simulink model "model_2_with_mpc"  (R2024a)
settings: Solver=VariableStepAuto  StartTime=0.0  StopTime=5  RelTol=1e-3
values from neighbouring files (symbols this model uses):
  d = 16.5e-2    (= 0.165)    [optParameters.m]
  fM = 8.108e-06    [optParameters.m]
  fw = 0.0047871    [optParameters.m]
  g = 9.8    [optParameters.m]
  JA = 0.00010012    [optParameters.m]
  JB = 0.01862    [optParameters.m]
  JM = 1.1538e-05    [optParameters.m]
  k = 43.8    [optParameters.m]
  kM = 0.0382    [optParameters.m]
  l = -0.02073    [optParameters.m]
  mb = 0.66855    [optParameters.m]
  mw = 53e-3    (= 0.053)    [optParameters.m]
  r = 3.25e-2    (= 0.0325)    [optParameters.m]
  R = 0.2    [load_example_QProblem.m]    (also in lqrandmpc.m = 0.1; optParameters.m = 16.696)
libraries: mpclib x1, aerolibutil x1, sharedutil x1, simulink_extras x1
settings Model: Creator=muham  LastModifiedBy=muham
settings RTWCC: GPUComputeCapability=3.5

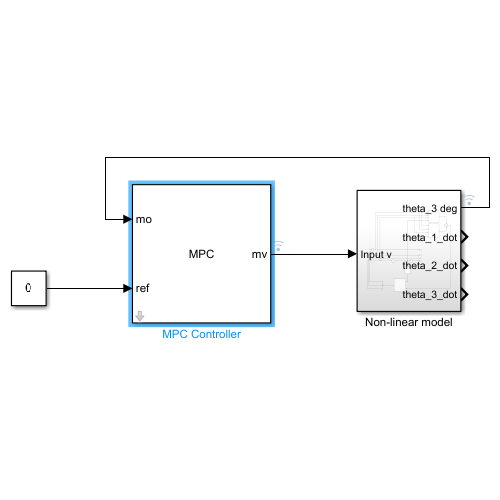
[thumbnail: Simulink's stored preview of the top-level diagram]
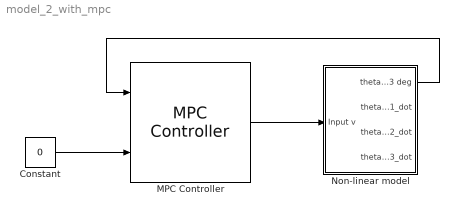
== system model_2_with_mpc ==
  Constant : Constant  Value=0
  MPC Controller : mpclib/MPC Controller  SCDEnableBlockLinearizationSpecification=on  mpcobj=mpc1  is_multiple=0  enable_value=0  return_u0=off  updateMPCinCallerWorkspace=on  md_inport=off  mv_inport=off  uref_inport=off  return_cost=off  return_mvseq=off  return_qpstatus=off  return_xseq=off  return_state=off  return_ovseq=off  state_inport=off  umin_inport=off  umax_inport=off  ymin_inport=off  ymax_inport=off  cc_inport=off  ywt_inport=off  uwt_inport=off  duwt_inport=off  rhoeps_inport=off  pm_inport=off  MaximumP=10  HorizonChoice=FixedHorizon  n_ts=0.01  n_p=40  n_mv=1  n_md=0  n_ud=0  n_mo=1  n_uo=0  BlockDataType=double  SampleTimeInherited=off  switch_inport=off
  Non-linear model : Subsystem
  wires:
  MPC Controller/1 -> Non-linear model/1(Input v)
  Constant/1 -> MPC Controller/2
  Non-linear model/1(theta_3 deg) -> MPC Controller/1

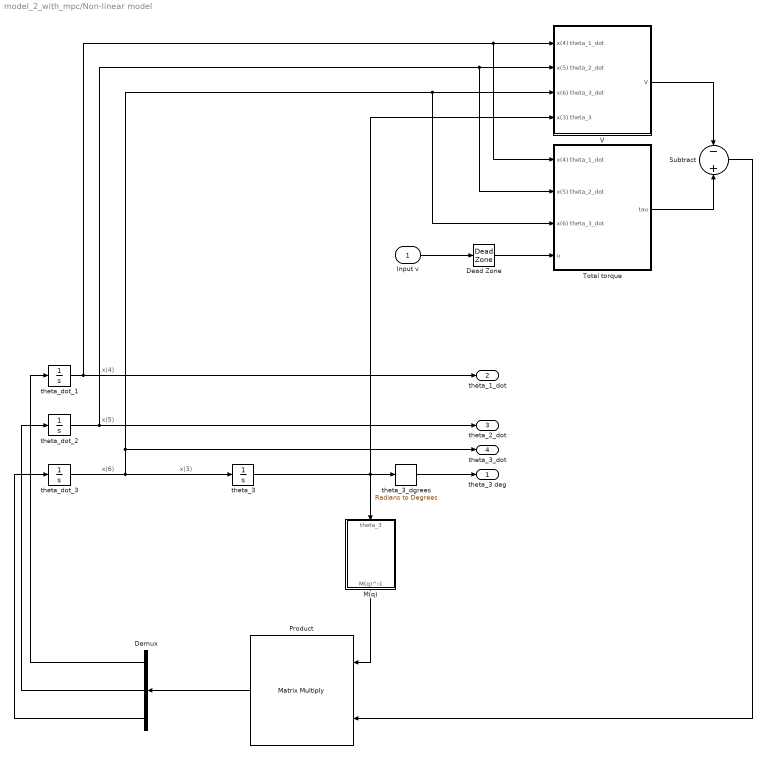
== system model_2_with_mpc/Non-linear model ==
  note: x(3)
  note: x(5)
  note: x(6)
  note: x(4)
  Input v : Inport
  Dead Zone : DeadZone  LowerValue=-1.5  UpperValue=1.5
  Demux : Demux  Outputs=3
  M(q) : Subsystem
  Product : Product  Multiplication=Matrix(*)
  Subtract : Sum  Inputs=-+
  Total torque : Subsystem
  V : Subsystem
  theta_3 : Integrator  WrappedStateUpperValue=pi/2  WrappedStateLowerValue=-pi/2
  theta_3_dgrees : simulink_extras/Transformations/Radians to Degrees
  theta_dot_1 : Integrator
  theta_dot_2 : Integrator
  theta_dot_3 : Integrator
  theta_3 deg : Outport
  theta_1_dot : Outport  Port=2
  theta_2_dot : Outport  Port=3
  theta_3_dot : Outport  Port=4
  wires:
  theta_dot_1/1 -> theta_1_dot/1, V/1(x(4) theta_1_dot), Total torque/1(x(4) theta_1_dot)
  theta_3/1 -> V/4(x(3) theta_3), theta_3_dgrees/1, M(q)/1(theta_3)
  Demux/3 -> theta_dot_3/1
  Demux/1 -> theta_dot_1/1
  Dead Zone/1 -> Total torque/4(u)
  theta_dot_3/1 -> Total torque/3(x(6) theta_3_dot), V/3(x(6) theta_3_dot), theta_3_dot/1, theta_3/1
  theta_3_dgrees/1 -> theta_3 deg/1
  M(q)/1(M(q)^-1) -> Product/1
  Product/1 -> Demux/1
  Subtract/1 -> Product/2
  theta_dot_2/1 -> theta_2_dot/1, V/2(x(5) theta_2_dot), Total torque/2(x(5) theta_2_dot)
  Total torque/1(tau) -> Subtract/2
  Input v/1 -> Dead Zone/1
  Demux/2 -> theta_dot_2/1
  V/1(V) -> Subtract/1

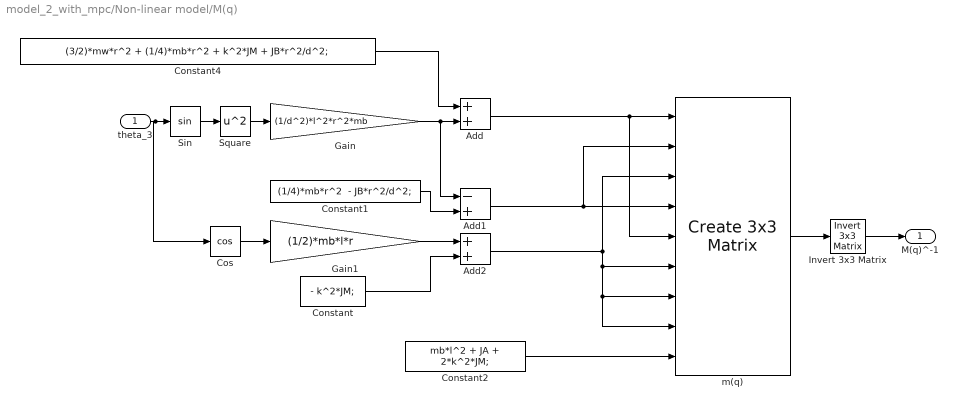
== system model_2_with_mpc/Non-linear model/M(q) ==
  theta_3 : Inport
  Add : Sum
  Add1 : Sum  Inputs=-+
  Add2 : Sum
  Constant : Constant  Value=- k^2*JM;
  Constant1 : Constant  Value="(1/4)*mb*r^2  - JB*r^2/d^2;"
  Constant2 : Constant  Value=mb*l^2 + JA + 2*k^2*JM;
  Constant4 : Constant  Value=(3/2)*mw*r^2 + (1/4)*mb*r^2 + k^2*JM + JB*r^2/d^2;
  Cos : Trigonometry  Operator=cos
  Gain : Gain  Gain=(1/d^2)*l^2*r^2*mb
  Gain1 : Gain  Gain=(1/2)*mb*l*r
  Invert 3x3 Matrix : aerolibutil/Invert  3x3 Matrix
  Sin : Trigonometry
  Square : Math  Operator=square
  m(q) : sharedutil/Create 3x3 Matrix  aMode=aMode
  M(q)^-1 : Outport
  wires:
  Cos/1 -> Gain1/1
  theta_3/1 -> Cos/1, Sin/1
  Gain/1 -> Add1/1, Add/2
  m(q)/1 -> Invert 3x3 Matrix/1
  Sin/1 -> Square/1
  Square/1 -> Gain/1
  Invert 3x3 Matrix/1 -> M(q)^-1/1
  Constant4/1 -> Add/1
  Add/1 -> m(q)/5, m(q)/1
  Add1/1 -> m(q)/2, m(q)/4
  Gain1/1 -> Add2/1
  Constant/1 -> Add2/2
  Add2/1 -> m(q)/3, m(q)/6, m(q)/8, m(q)/7
  Constant2/1 -> m(q)/9
  Constant1/1 -> Add1/2

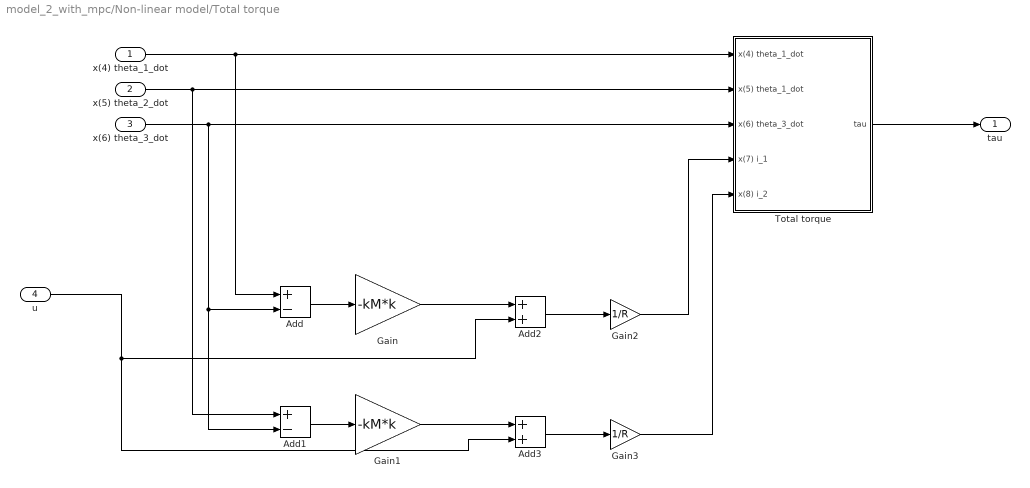
== system model_2_with_mpc/Non-linear model/Total torque ==
  x(4) theta_1_dot : Inport
  x(5) theta_2_dot : Inport  Port=2
  x(6) theta_3_dot : Inport  Port=3
  u : Inport  Port=4
  Add : Sum  Inputs=+-
  Add1 : Sum  Inputs=+-
  Add2 : Sum
  Add3 : Sum
  Gain : Gain  Gain=-kM*k
  Gain1 : Gain  Gain=-kM*k
  Gain2 : Gain  Gain=1/R
  Gain3 : Gain  Gain=1/R
  Total torque : Subsystem
  tau : Outport
  wires:
  x(6) theta_3_dot/1 -> Add1/2, Add/2, Total torque/3(x(6) theta_3_dot)
  x(5) theta_2_dot/1 -> Add1/1, Total torque/2(x(5) theta_1_dot)
  x(4) theta_1_dot/1 -> Add/1, Total torque/1(x(4) theta_1_dot)
  Total torque/1(tau) -> tau/1
  Add/1 -> Gain/1
  Add1/1 -> Gain1/1
  Add2/1 -> Gain2/1
  u/1 -> Add3/2, Add2/2
  Gain/1 -> Add2/1
  Gain2/1 -> Total torque/4(x(7) i_1)
  Add3/1 -> Gain3/1
  Gain3/1 -> Total torque/5(x(8) i_2)
  Gain1/1 -> Add3/1

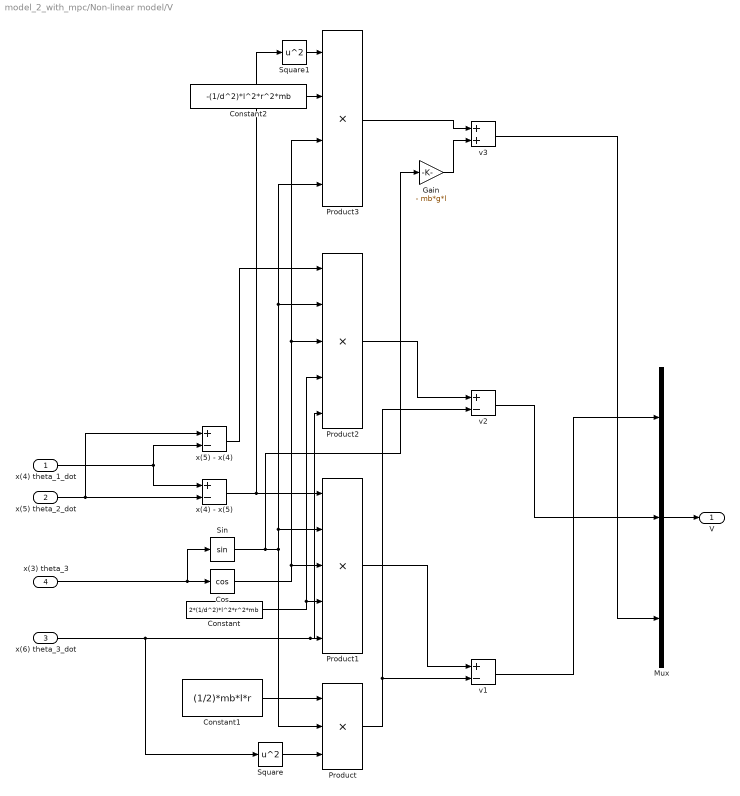
== system model_2_with_mpc/Non-linear model/V ==
  x(4) theta_1_dot : Inport
  x(5) theta_2_dot : Inport  Port=2
  x(6) theta_3_dot : Inport  Port=3
  x(3) theta_3 : Inport  Port=4
  Constant : Constant  Value=2*(1/d^2)*l^2*r^2*mb
  Constant1 : Constant  Value=(1/2)*mb*l*r
  Constant2 : Constant  Value=-(1/d^2)*l^2*r^2*mb
  Cos : Trigonometry  Operator=cos
  Gain : Gain  Gain=- mb*g*l
  Mux : Mux  Inputs=3
  Product : Product  Inputs=3
  Product1 : Product  Inputs=5
  Product2 : Product  Inputs=5
  Product3 : Product  Inputs=4
  Sin : Trigonometry
  Square : Math  Operator=square
  Square1 : Math  Operator=square
  v1 : Sum  Inputs=+-
  v2 : Sum  Inputs=+-
  v3 : Sum
  x(4) - x(5) : Sum  Inputs=+-
  x(5) - x(4) : Sum  Inputs=+-
  V : Outport
  wires:
  x(5) theta_2_dot/1 -> x(4) - x(5)/2, x(5) - x(4)/1
  x(3) theta_3/1 -> Cos/1, Sin/1
  x(4) theta_1_dot/1 -> x(4) - x(5)/1, x(5) - x(4)/2
  Constant/1 -> Product2/4, Product1/4
  x(6) theta_3_dot/1 -> Product2/5, Product1/5, Square/1
  x(4) - x(5)/1 -> Product1/1, Square1/1
  Cos/1 -> Product3/3, Product2/3, Product1/3
  Product1/1 -> v1/1
  Constant1/1 -> Product/1
  Product/1 -> v2/2, v1/2
  Square/1 -> Product/3
  x(5) - x(4)/1 -> Product2/1
  Sin/1 -> Gain/1, Product3/4, Product2/2, Product1/2, Product/2
  Product2/1 -> v2/1
  Constant2/1 -> Product3/2
  Square1/1 -> Product3/1
  Product3/1 -> v3/1
  Gain/1 -> v3/2
  v1/1 -> Mux/1
  v2/1 -> Mux/2
  v3/1 -> Mux/3
  Mux/1 -> V/1

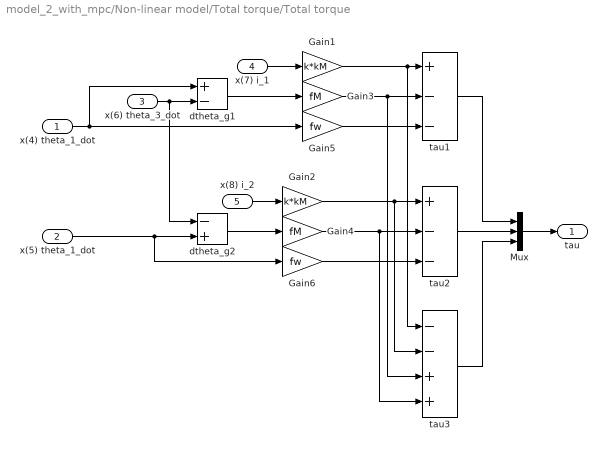
== system model_2_with_mpc/Non-linear model/Total torque/Total torque ==
  x(4) theta_1_dot : Inport
  x(5) theta_1_dot : Inport  Port=2
  x(6) theta_3_dot : Inport  Port=3
  x(7) i_1 : Inport  Port=4
  x(8) i_2 : Inport  Port=5
  Gain1 : Gain  Gain=k*kM
  Gain2 : Gain  Gain=k*kM
  Gain3 : Gain  Gain=fM
  Gain4 : Gain  Gain=fM
  Gain5 : Gain  Gain=fw
  Gain6 : Gain  Gain=fw
  Mux : Mux  Inputs=3
  dtheta_g1 : Sum  Inputs=+-
  dtheta_g2 : Sum  Inputs=-+
  tau1 : Sum  Inputs=+--
  tau2 : Sum  Inputs=+--
  tau3 : Sum  Inputs=--++
  tau : Outport
  wires:
  Gain6/1 -> tau2/3
  Gain3/1 -> tau1/2, tau3/3
  Gain1/1 -> tau3/1, tau1/1
  Gain5/1 -> tau1/3
  Gain2/1 -> tau3/2, tau2/1
  x(4) theta_1_dot/1 -> Gain5/1, dtheta_g1/1
  Gain4/1 -> tau3/4, tau2/2
  dtheta_g2/1 -> Gain4/1
  tau1/1 -> Mux/1
  dtheta_g1/1 -> Gain3/1
  x(5) theta_1_dot/1 -> dtheta_g2/2, Gain6/1
  x(7) i_1/1 -> Gain1/1
  x(6) theta_3_dot/1 -> dtheta_g2/1, dtheta_g1/2
  x(8) i_2/1 -> Gain2/1
  tau2/1 -> Mux/2
  tau3/1 -> Mux/3
  Mux/1 -> tau/1
